simulink model "Huginn"  (R2024b)
settings: Solver=FixedStepAuto  StartTime=0.0  StopTime=525  FixedStep=0.1  RelTol=1e-3
model workspace (MAT data in the model file):
  N_P0 = 3
  fuel_map = [8.33e-06 8.33e-06 8.33e-06 8.33e-06 8.33e-06 8.33e-06 8.33e-06 8.33e-06 8.33e-06 8.33e-06 8.33e-06 8.33e-06 ... (2082 elements, 1041x2)]
  rpm_bp = [0 10 20 30 40 50 60 70 80 90 100 110 ... (671 elements, 671x1)]
  rpm_bp_fuel = [1200 1210 1220 1230 1240 1250 1260 1270 1280 1290 1300 1310 ... (1041 elements, 1041x1)]
  throttle_bp = [0 10 20 30 40 50 60 70 80 90 100]
  throttle_bp_fuel = [0; 1]
  torque_bp = [0.332105118453 0.337426322834 0.342845115066 0.348363542915 0.353983594259 0.359707194633 0.36553620448 0.371483133692 0.377549913828 0.383738457661 0.390050655328 0.396488370473 ... (901 elements, 901x1)]
  torque_map = [0 0 0 0 0 0 0 0 0 0 0 0 ... (7381 elements, 671x11)]
values from neighbouring files (symbols this model uses):
  rpm_fine = [1200 1210 1220 1230 1240 1250 1260 1270 1280 1290 1300 1310 ... (1041 elements, 1041x1)]    [optimised workspace.mat]    (also in run_before_huginn.m = (min(rpm_bp) : 10 : max(rpm_bp))')
  throttle_fine = [0 1]    [optimised workspace.mat]    (also in run_before_huginn.m = (min(throttle_bp) : 1 : max(throttle_bp))')
  throttle_profile = [14.9858312924 0 60 60 60 0.55631746946 8.17065947955 1.9881415447 9.75633320207 0.0428601079869 58.2417871472 60 ... (25 elements, 1x25)]    [Optimised_fuel_2.mat]    (also in optimised workspace.mat = [65.5401746966 57.4724229506 57.2057862197 67.539022656 57.9; other optmised.mat)
undefined symbols (not defined in the file or in its folder): DiscIntNeverNeededParam, dspblkCoreblockFVToolHelper, gcbh
(part 1 of 2)
settings Model: Creator=Pain  LastModifiedBy=Pain
settings DataIOCC: ReturnWorkspaceOutputsName=SDOSimTest_Log

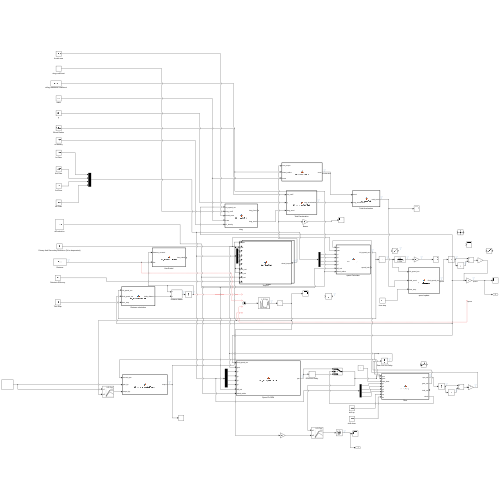
[thumbnail: Simulink's stored preview of the top-level diagram]
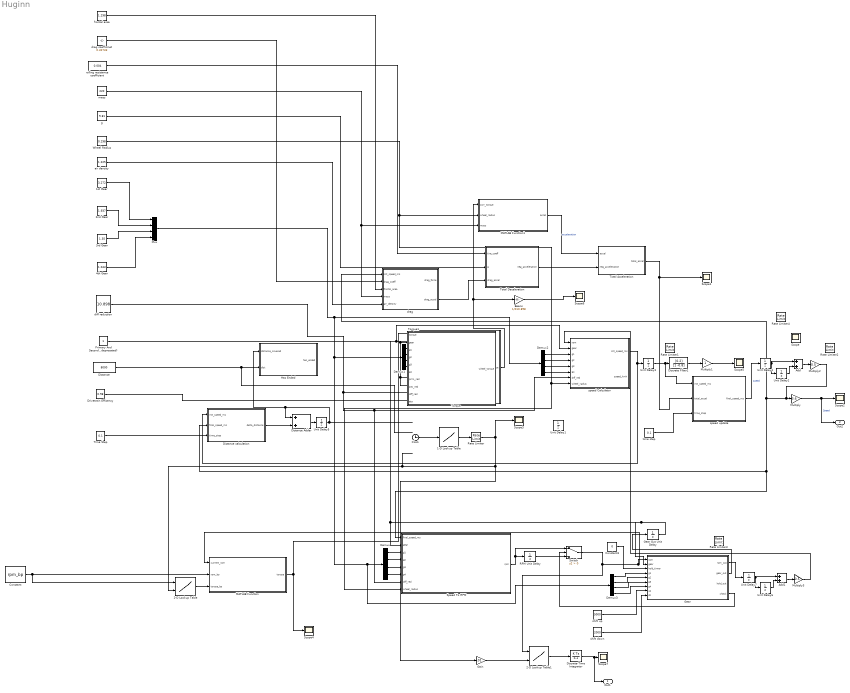
== system Huginn ==
  1-D Lookup Table : Lookup_n-D  NumberOfTableDimensions=1  BreakpointsForDimension1=linspace(0, 525, length(throttle_profile))  Table=throttle_profile  ExtrapMethod=Clip  InternalRulePriority=Speed  RndMeth=Simplest
  1st Gear : Constant  Value=3.272
  2-D Lookup Table : Lookup_n-D  BreakpointsForDimension1=rpm_bp  BreakpointsForDimension2=throttle_bp  Table=torque_map  ExtrapMethod=Clip  InternalRulePriority=Speed  RndMeth=Simplest
      settings: InputPortMap=u0,u1
  2-D Lookup Table1 : Lookup_n-D  BreakpointsForDimension1=rpm_fine  BreakpointsForDimension2=throttle_fine  Table=fuel_map  InternalRulePriority=Speed  RndMeth=Simplest
      settings: InputPortMap=u0,u1
  2nd Gear : Constant  Value=1.937
  3rd Gear : Constant  Value=1.35
  4th Gear : Constant  Value=1.043
  Add : Sum
  Add1 : Sum
  Beans : Gain  Gain=1/010.898
  Clock : Clock
  Constant : Constant  Value=rpm_bp
  Constant3 : Constant  Value=0
  Demux{,1..3} (4 alike) : Demux
  Discrete Filter1 : DiscreteFilter  LoadFcn=dspblkCoreblockFVToolHelper(gcbh,'load');  Numerator=[0.2]  Denominator=[1 -0.8]
      settings: CopyFcn=dspblkCoreblockFVToolHelper(gcbh,'copy');  DeleteFcn=dspblkCoreblockFVToolHelper(gcbh,'close');  ModelCloseFcn=dspblkCoreblockFVToolHelper(gcbh,'close');  PreSaveFcn=dspblkCoreblockFVToolHelper(gcbh,'presave');  PostSaveFcn=dspblkCoreblockFVToolHelper(gcbh,'postsave');  CloseFcn=dspblkCoreblockFVToolHelper(gcbh,'close');
  Discrete-Time Integrator : DiscreteIntegrator  SampleTime=-1  ICPrevOutput=DiscIntNeverNeededParam  ICPrevScaledInput=DiscIntNeverNeededParam
  Distance : Constant  Value=8000
  Distance Adder : Sum
  Distance calculation : MATLAB Function  TreatAsAtomicUnit=on
  Drivetrain Efficency : Constant  Value=0.98
  Gain : Gain  Gain=.01
  Gear : MATLAB Function  TreatAsAtomicUnit=on
  Gear Out Unit Delay : UnitDelay  InitialCondition=1  SampleTime=0.5  HasFrameUpgradeWarning=on
  Has Ended : MATLAB Function  TreatAsAtomicUnit=on
  MATLAB Function : MATLAB Function  TreatAsAtomicUnit=on
  MATLAB Function1 : MATLAB Function  TreatAsAtomicUnit=on
  Multiply : Gain  Gain=3.6
  Multiply1 : Gain
  Multiply2 : Gain  Gain=0.5
  Multiply3 : Gain  Gain=0.5
  Mux : Mux
  Primary And Secondary Reduction (To be deprecated) : Constant
  RPM Unit Delay : UnitDelay  InitialCondition=4500  SampleTime=0.1  HasFrameUpgradeWarning=on
  Rate Limiter : RateLimiter  RisingSlewLimit=5  FallingSlewLimit=-5  SampleTimeMode=inherited
  Rate Limiter1 : RateLimiter  RisingSlewLimit=7  FallingSlewLimit=-7  SampleTimeMode=inherited
  Rate Limiter2 : RateLimiter  RisingSlewLimit=5  FallingSlewLimit=-5  SampleTimeMode=inherited
  Rate Limiter3 : RateLimiter  RisingSlewLimit=5  FallingSlewLimit=-5  SampleTimeMode=inherited
  Rate Limiter4 : RateLimiter  RisingSlewLimit=7  FallingSlewLimit=-7  SampleTimeMode=inherited
  Scope{,1..7} (8 alike) : Scope
  Speed To RPM : MATLAB Function  TreatAsAtomicUnit=on
  Switch : Switch  Criteria=u2 > Threshold  SaturateOnIntegerOverflow=off  InputSameDT=off
  Time Step : Constant  Value=0.1
  Torque : MATLAB Function  TreatAsAtomicUnit=on
  Torque1 : MATLAB Function  TreatAsAtomicUnit=on
  Total Acceleration : MATLAB Function  TreatAsAtomicUnit=on
  Total Deceleration : MATLAB Function  TreatAsAtomicUnit=on
  Unit Delay1 : UnitDelay  SampleTime=-1  HasFrameUpgradeWarning=on
  Unit Delay2 : UnitDelay  InitialCondition=8.99  SampleTime=0.1  HasFrameUpgradeWarning=on
  Unit Delay3 : UnitDelay  InitialCondition=1  InputProcessing=Columns as channels (frame based)  SampleTime=0.1  HasFrameUpgradeWarning=on
  Unit Delay4 : UnitDelay  InitialCondition=8.99  SampleTime=0.1  HasFrameUpgradeWarning=on
  Unit Delay5 : UnitDelay  SampleTime=-1  HasFrameUpgradeWarning=on
  Unit Delay6 : UnitDelay  InitialCondition=4500  SampleTime=0.1  HasFrameUpgradeWarning=on
  Unit Delay7 : UnitDelay  InitialCondition=4500  SampleTime=0.1  HasFrameUpgradeWarning=on
  Wheel Radius : Constant  Value=0.298
  air density : Constant  Value=1.225
  diff reduction : Constant  Value=10.898
  drag : MATLAB Function  TreatAsAtomicUnit=on
  drag coefficinet : Constant  Value=0.32733
  frontal area : Constant  Value=1.298
  g : Constant  Value=9.81
  mass : Constant  Value=220
  rolling resistance coefficient : Constant  Value=0.004
  shift down : Constant  Value=2000
  shift up : Constant  Value=5000
  speed Calculator : MATLAB Function  TreatAsAtomicUnit=on
  speed update : MATLAB Function  TreatAsAtomicUnit=on
  time step : Constant  Value=0.1
  Out1 : Outport
  Out2 : Outport  Port=2
  wires:
  Distance/1 -> Has Ended/2(dist)
  Constant/1 -> 2-D Lookup Table/1, MATLAB Function/2(rpm_bp)
  2-D Lookup Table/1 -> MATLAB Function/3(torque_bp)
  Total Deceleration/1(neg_acceleration) -> Total Acceleration/2(neg_acceleration)
  Distance calculation/1(delta_distance) -> Distance Adder/2
  Unit Delay5/1 -> Has Ended/1(distance_covered), Distance Adder/1
  Multiply2/1 -> Speed To RPM/1(final_speed_ms), Distance calculation/2(final_speed_ms), drag/1(init_speed_ms), Multiply/1
  ? -> ?  "Speed"
  speed Calculator/1(init_speed_ms) -> Unit Delay3/1, Distance calculation/1(init_speed_ms)
  Total Acceleration/1(total_accel) -> speed update/2(total_accel), Scope1/1
  MATLAB Function/1(torque) -> Scope4/1, Torque/1(torque)
  Torque/1(wheel_torque) -> Beans/1, MATLAB Function1/1(corr_torque)
  MATLAB Function1/1(accel) -> Total Acceleration/1(accel)  "acceleration"
  Multiply3/1 -> speed Calculator/1(rpm)
  Time Step/1 -> Distance calculation/3(time_step)
  Primary And Secondary Reduction (To be deprecated)/1 -> Torque1/2(gear), Torque/8(sec_red), Torque/7(prim_red)
  Drivetrain Efficency/1 -> Torque/10(eta)
  Gear/2(gear_out) -> Gear Out Unit Delay/1
  1st Gear/1 -> Mux/1
  2nd Gear/1 -> Mux/2
  3rd Gear/1 -> Mux/3
  4th Gear/1 -> Mux/4
  Demux/1 -> Speed To RPM/3(g1)
  Demux/2 -> Speed To RPM/4(g2)
  Demux/3 -> Speed To RPM/5(g3)
  Demux/4 -> Speed To RPM/6(g4)
  Demux1/1 -> Torque/3(g1)
  Demux1/2 -> Torque/4(g2)
  Demux1/3 -> Torque/5(g3)
  Demux1/4 -> Torque/6(g4)
  Demux2/1 -> speed Calculator/3(g1)
  Demux2/2 -> speed Calculator/4(g2)
  Demux2/3 -> speed Calculator/5(g3)
  Demux2/4 -> speed Calculator/6(g4)
  Mux/1 -> Demux2/1, Demux3/1, Demux/1, Demux1/1
  Demux3/1 -> Gear/4(g1)
  Demux3/2 -> Gear/5(g2)
  Demux3/3 -> Gear/6(g3)
  Demux3/4 -> Gear/7(g4)
  diff reduction/1 -> Speed To RPM/7(diff_red), speed Calculator/7(diff_red), Torque/9(diff_red)
  g/1 -> Total Deceleration/2(g)
  mass/1 -> drag/4(mass), MATLAB Function1/3(mass)
  rolling resistance coefficient/1 -> Total Deceleration/1(tire_coeff)
  air density/1 -> drag/5(air_density)
  drag coefficinet/1 -> drag/2(drag_coeff)
  frontal area/1 -> drag/3(frontal_area)
  shift up/1 -> Gear/8(up)
  shift down/1 -> Gear/9(dn)
  Gear Out Unit Delay/1 -> Gear/2(gear), Speed To RPM/2(gear), Torque/2(gear), speed Calculator/2(gear)
  drag/2(drag_accel) -> Total Deceleration/3(drag_accel)
  Switch/1 -> 2-D Lookup Table1/1, MATLAB Function/1(current_rpm), Gear/1(rpm)
  Distance Adder/1 -> Unit Delay5/1
  Unit Delay3/1 -> speed update/1(init_speed_ms), Discrete Filter1/1
  speed update/1(final_speed_ms) -> Unit Delay4/1  "speed"
  1-D Lookup Table/1 -> Rate Limiter/1
  time step/1 -> speed update/3(time_step)
  Wheel Radius/1 -> Speed To RPM/8(wheel_radius), speed Calculator/8(wheel_radius), MATLAB Function1/2(wheel_radius)
  Rate Limiter/1 -> Gain/1, 2-D Lookup Table/2, Scope3/1
  Discrete Filter1/1 -> Multiply1/1
  Multiply1/1 -> Scope5/1
  Unit Delay4/1 -> Unit Delay2/1, Add/1
  Unit Delay2/1 -> Add/2
  Add/1 -> Multiply2/1
  Speed To RPM/1(rpm) -> Switch/1, RPM Unit Delay/1
  Beans/1 -> Scope6/1
  Unit Delay7/1 -> Unit Delay6/1, Add1/1
  Add1/1 -> Multiply3/1
  Unit Delay6/1 -> Add1/2
  Gear/1(rpm_out) -> Unit Delay7/1
  Constant3/1 -> Gear/3(hold_timer)
  RPM Unit Delay/1 -> Switch/3
  Gear/4(check) -> Switch/2
  2-D Lookup Table1/1 -> Discrete-Time Integrator/1
  Discrete-Time Integrator/1 -> Out1/1, Scope7/1
  Gain/1 -> 2-D Lookup Table1/2
  Clock/1 -> 1-D Lookup Table/1
  Multiply/1 -> Out2/1, Scope2/1  "Speed"
